simulink model "Question_3"  (R2024b)
settings: Solver=VariableStepAuto  StartTime=0.0  StopTime=10.0  RelTol=1e-3
model workspace (MAT data in the model file):
  LIGHT = 0
  LightSignal = 0
settings Model: Creator=Sagar  LastModifiedBy=Sagar

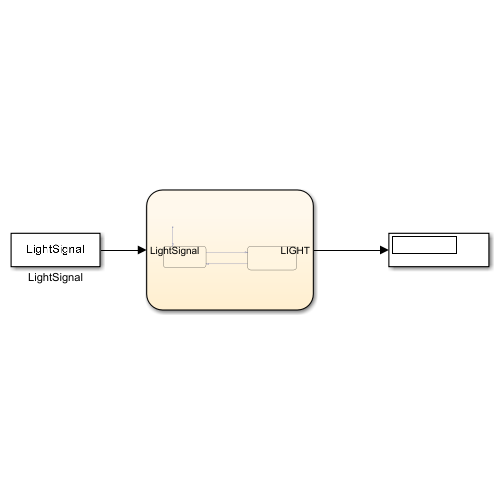
[thumbnail: Simulink's stored preview of the top-level diagram]
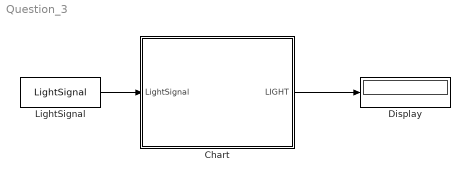
== system Question_3 ==
  Chart : Stateflow chart  TreatAsAtomicUnit=on
  Display : Display
  LightSignal : Constant  Value=LightSignal
  wires:
  LightSignal/1 -> Chart/1(LightSignal)
  Chart/1(LIGHT) -> Display/1

== stateflow chart Question_3/Chart ==
  state ON
    entry:
    LIGHT=1
    disp('LightState: ON')
  state OFF
    entry:
    LIGHT= 0
    disp('LightState: OFF ')
  (default) -> ON
  ON -> OFF : [LightSignal == 0]
  OFF -> ON : [LightSignal ==1]
  data: LightSignal input; LIGHT output
